simulink model "assignment9_1_model"  (R2024b)
settings: Solver=VariableStepAuto  StartTime=0.0  StopTime=10.0  RelTol=1e-3

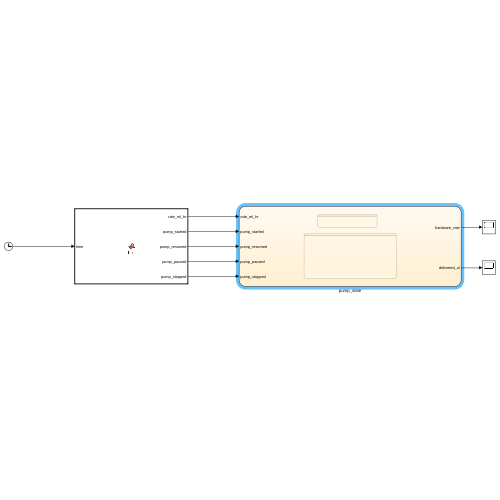
[thumbnail: Simulink's stored preview of the top-level diagram]
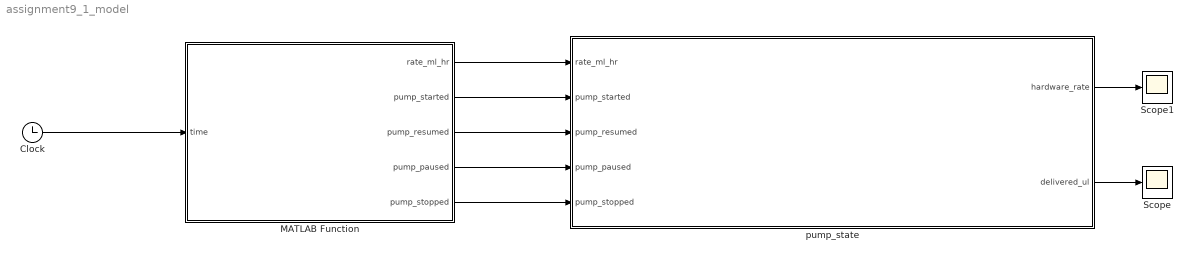
== system assignment9_1_model ==
  Clock : Clock
  MATLAB Function : MATLAB Function  TreatAsAtomicUnit=on
  Scope : Scope
  Scope1 : Scope
  pump_state : Stateflow chart  TreatAsAtomicUnit=on
  wires:
  pump_state/1(hardware_rate) -> Scope1/1
  Clock/1 -> MATLAB Function/1(time)
  MATLAB Function/1(rate_ml_hr) -> pump_state/1(rate_ml_hr)
  MATLAB Function/4(pump_paused) -> pump_state/4(pump_paused)
  MATLAB Function/3(pump_resumed) -> pump_state/3(pump_resumed)
  MATLAB Function/5(pump_stopped) -> pump_state/5(pump_stopped)
  MATLAB Function/2(pump_started) -> pump_state/2(pump_started)
  pump_state/2(delivered_ul) -> Scope/1

== matlab function assignment9_1_model/MATLAB Function ==
  data: time input; rate_ml_hr output; pump_started output; pump_resumed output; pump_paused output; pump_stopped output
function [rate_ml_hr, pump_started, pump_resumed, pump_paused, pump_stopped] = fcn(time)
% time is in seconds, like from a Simulink Clock block

  step_size = 0.1;  % one time step every 0.1 seconds

  test_cases = [
  600, 1, 0, 0, 0;  % t=0.0: stop pulse (reset FSM)
  600, 1, 0, 0, 0;  % t=0.1: settle
  600, 1, 0, 0, 0;  % t=0.2: start pulse
  600, 0, 0, 0, 0;  % t=0.3: settle
  600, 0, 0, 1, 0;  % t=0.4: pause pulse
  600, 0, 0, 0, 0;  % t=0.5: settle
  600, 0, 0, 0, 1;  % t=0.6: resume pulse
  600, 0, 0, 0, 0;  % t=0.7: settle
  600, 0, 0, 1, 0;  % t=0.8: pause pulse again
  600, 0, 0, 0, 0;  % t=0.9: settle
  600, 0, 1, 0, 0;  % t=1.0: stop pulse again
  600, 0, 0, 0, 0;  % t=1.1: end
  600, 1, 0, 0, 0;  % t=0.0: stop pulse (reset FSM)
  600, 1, 0, 0, 0;  % t=0.0: stop pulse (reset FSM)
  600, 0, 1, 0, 0;  % t=0.0: stop pulse (reset FSM)
];

  % Convert time into an index (1-based)
  idx = floor(time / step_size) + 1;

  % Clamp to valid range
  idx = min(max(1, idx), size(test_cases, 1));

  % Extract values
  rate_ml_hr    = uint32(test_cases(idx, 1));
  pump_started  = logical(test_cases(idx, 2));
  pump_resumed  = logical(test_cases(idx, 5));
  pump_paused   = logical(test_cases(idx, 4));
  pump_stopped  = logical(test_cases(idx, 3));

  % Optional: Console log (won’t appear during codegen or accelerator mode)
  if ~coder.target('RTW')  % only run in normal simulation
  fprintf('t=%.1f -> rate=%u, start=%d, stop=%d, pause=%d, resume=%d\n', ...
    time, rate_ml_hr, ...
    int8(pump_started), int8(pump_stopped), int8(pump_paused), int8(pump_resumed));
  end
end

== stateflow chart assignment9_1_model/pump_state ==
  state MotorState [parallel]
    settings: executionOrder=1
    state Off
      entry:
      motor_on = false;
    state On
      entry:
      motor_on = true;
    (default) -> Off
    Off -> On : [pump_started || pump_resumed]
    On -> Off : [pump_paused || pump_stopped]
  state PumpState [parallel]
    settings: executionOrder=2
    state Idle
    state Infusing
    state PumpError
    state Paused
    Infusing -> PumpError [order 3] : [pump_resumed]
    (default) -> Idle
    Idle -> Infusing [order 1] : [pump_started && rate_ml_hr > 0]
        | {delivered_ul = 0;
        | hardware_rate = rate_ml_hr;}
    Idle -> PumpError [order 2] : [pump_stopped]
    Infusing -> Idle [order 1] : [pump_stopped]
    Paused -> Idle [order 2] : [pump_stopped]
    Paused -> Infusing [order 1] : [pump_resumed]
    Infusing -> Paused [order 2] : [pump_paused]
    Paused -> PumpError [order 3] : [pump_paused || pump_started]
  data: rate_ml_hr input; pump_started input; pump_resumed input; pump_paused input; hardware_rate output; motor_on local; delivered_ul output; pump_stopped input
